simulink model "car"  (Simulink 8.7)
settings: Solver=ode45  StartTime=0.0  StopTime=200  FixedStep=0.01  RelTol=1e-3
libraries: Solver_SF x1
settings Model: Creator=xuwei  LastModifiedBy=Gyl
settings DataIOCC: SignalLoggingSaveFormat=ModelDataLogs
settings OptimizationCC: ExpressionDepthLimit=2147483647
settings DebuggingCC: SolverPrmCheckMsg=warning  FcnCallInpInsideContextMsg=EnableAllAsWarning  StateNameClashWarn=warning  StrictBusMsg=Warning
settings GRTTargetCC: CombineOutputUpdateFcns=off  GRTInterface=on
settings ConfigComp: CovModelRefEnable=off

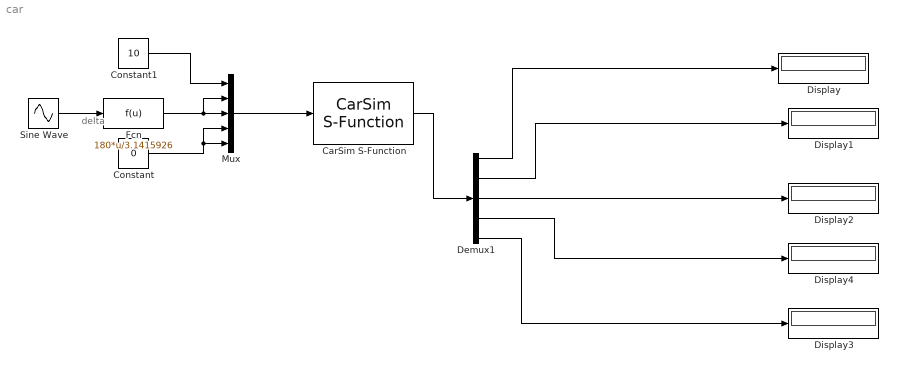
== system car ==
  note: delta
  CarSim S-Function : Solver_SF/CarSim S-Function  Priority=1  VehicleCode=i_i  SIMFILE=simfile.sim
  Constant : Constant  Value=0
  Constant1 : Constant  Value=10
  Demux1 : Demux  Outputs=5
  Display{,1..4} (5 alike) : Display
  Fcn : Fcn  Expr=180*u/3.1415926
  Mux : Mux  Inputs=5
  Sine Wave : Sin  Amplitude=0.2  Frequency=5  SampleTime=0
  wires:
  CarSim S-Function/1 -> Demux1/1
  Mux/1 -> CarSim S-Function/1
  Demux1/1 -> Display/1
  Demux1/2 -> Display1/1
  Demux1/3 -> Display2/1
  Demux1/4 -> Display4/1
  Demux1/5 -> Display3/1
  Fcn/1 -> Mux/2, Mux/3
  Constant/1 -> Mux/4, Mux/5
  Constant1/1 -> Mux/1
  Sine Wave/1 -> Fcn/1
